simulink model "model_kalman_filter"  (R2022a)
settings: Solver=ode23t  StartTime=0.0  StopTime=0.1  FixedStep=0.001  RelTol=1e-3
undefined symbols (not defined in the file or in its folder): A, B, C, Const_input, D, Kr, x_des
settings Model: Creator=asmax  LastModifiedBy=asmax
settings SolverCC: EnableFixedStepZeroCrossing=on

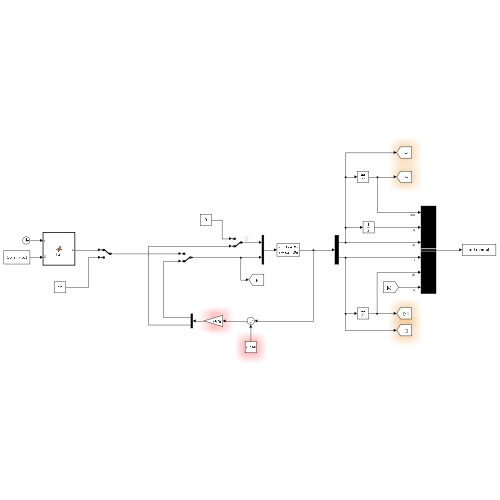
[thumbnail: Simulink's stored preview of the top-level diagram]
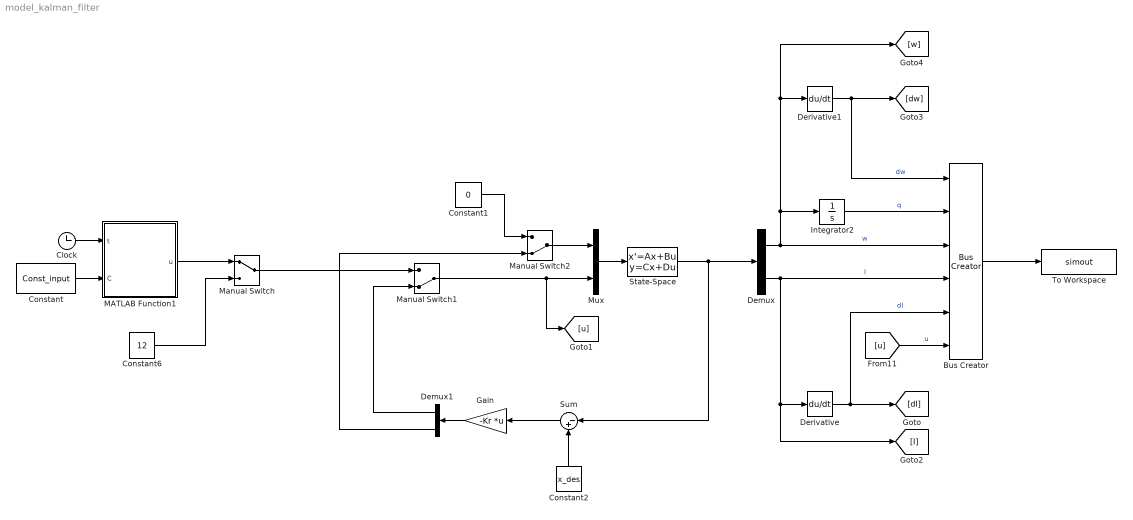
== system model_kalman_filter ==
  Bus Creator : BusCreator  Inputs=6
  Clock : Clock
  Constant : Constant  Value=Const_input
  Constant1 : Constant  Value=0
  Constant2 : Constant  Value=x_des
  Constant6 : Constant  Value=12
  Demux : Demux  Outputs=2
  Demux1 : Demux  Outputs=2
  Derivative : Derivative
  Derivative1 : Derivative
  Gain : Gain  Gain=-Kr  Multiplication=Matrix(K*u)
  Integrator2 : Integrator
  MATLAB Function1 : MATLAB Function  TreatAsAtomicUnit=on
  Manual Switch : ManualSwitch
  Manual Switch1 : ManualSwitch  CurrentSetting=0
  Manual Switch2 : ManualSwitch  CurrentSetting=0
  Mux : Mux  Inputs=2
  State-Space : StateSpace  A=A  B=B  C=C  D=D  InitialCondition=[0;0]
  Sum : Sum  Inputs=|-+
  To Workspace : ToWorkspace  VariableName=simout  SaveFormat=Timeseries  SampleTime=-1
  wires:
  Mux/1 -> State-Space/1
  State-Space/1 -> Sum/1, Demux/1
  Demux/1 -> Integrator2/1, [w], Derivative1/1, Bus Creator/3  "w"
  Demux/2 -> [I], Derivative/1, Bus Creator/4  "I"
  Bus Creator/1 -> To Workspace/1
  Derivative/1 -> Bus Creator/5, [dI]  "dI"
  Derivative1/1 -> [dw], Bus Creator/1  "dw"
  Clock/1 -> MATLAB Function1/1(t)
  MATLAB Function1/1(u) -> Manual Switch/1
  Constant6/1 -> Manual Switch/2
  Integrator2/1 -> Bus Creator/2  "q"
  [u] -> Bus Creator/6  "u"
  Constant/1 -> MATLAB Function1/2(C)
  Manual Switch/1 -> Manual Switch1/1
  Manual Switch1/1 -> [u], Mux/2
  Gain/1 -> Demux1/1
  Sum/1 -> Gain/1
  Constant2/1 -> Sum/2
  Demux1/1 -> Manual Switch1/2
  Demux1/2 -> Manual Switch2/2
  Manual Switch2/1 -> Mux/1
  Constant1/1 -> Manual Switch2/1

== matlab function model_kalman_filter/MATLAB Function1 ==
  data: t input; u output; C input
function u = fcn(t, C)

% w = 4;
% A = 6;
% B = 6;
% fi = 3.1415;
% u = A * cos(w * t + fi) + B;

w = C(3);
A = C(1);
B = C(2);
fi = C(4);
u = A * cos(w * t + fi) + B;
